simulink model "reglersystem"  (R2017a)
settings: Solver=FixedStepAuto  StartTime=0.0  StopTime=inf  RelTol=1e-3
libraries: robotlib x9, simulink x2
settings Model: Creator=simonpersson  LastModifiedBy=simonpersson
settings OptimizationCC: PassReuseOutputArgsAs=Individual arguments  MaxStackSize=64
settings DebuggingCC: ParameterTunabilityLossMsg=error
settings HardwareCC: ProdBitPerPointer=32  ProdBitPerSizeT=32  ProdBitPerPtrDiffT=32  ProdLargestAtomicFloat=None  ProdIntDivRoundTo=Undefined  ProdEndianess=Unspecified  ProdWordSize=32  ProdHWDeviceType=Generic->Unspecified (assume 32-bit Generic)
settings SFSimCC: MATLABDynamicMemAlloc=off
settings RTWCC: SystemTargetFile=ert.tlc  HardwareBoard=Robot Operating System (ROS)  TLCOptions="-aInlineSetEventsForThisBaseRateFcn=TLC_FALSE -aSuppressMultiTaskScheduler=TLC_FALSE  -aRateBasedStepFcn=0"  TemplateMakefile=ert_default_tmf  Description=Embedded Coder  GenerateReport=on  Toolchain=Catkin  IncludeHyperlinkInReport=on  LaunchReport=on  TargetLang=C++  GenerateTraceInfo=on  GenerateTraceReport=on  GenerateTraceReportSl=on  GenerateTraceReportSf=on  GenerateTraceReportEml=on
settings CodeAppCC: ForceParamTrailComments=on  IgnoreCustomStorageClasses=off  OperatorAnnotations=on  SimulinkDataObjDesc=on  SFDataObjDesc=on  MATLABFcnDesc=on  InsertBlockDesc=on  MATLABSourceComments=on
settings ERTTargetCC: SupportContinuousTime=on

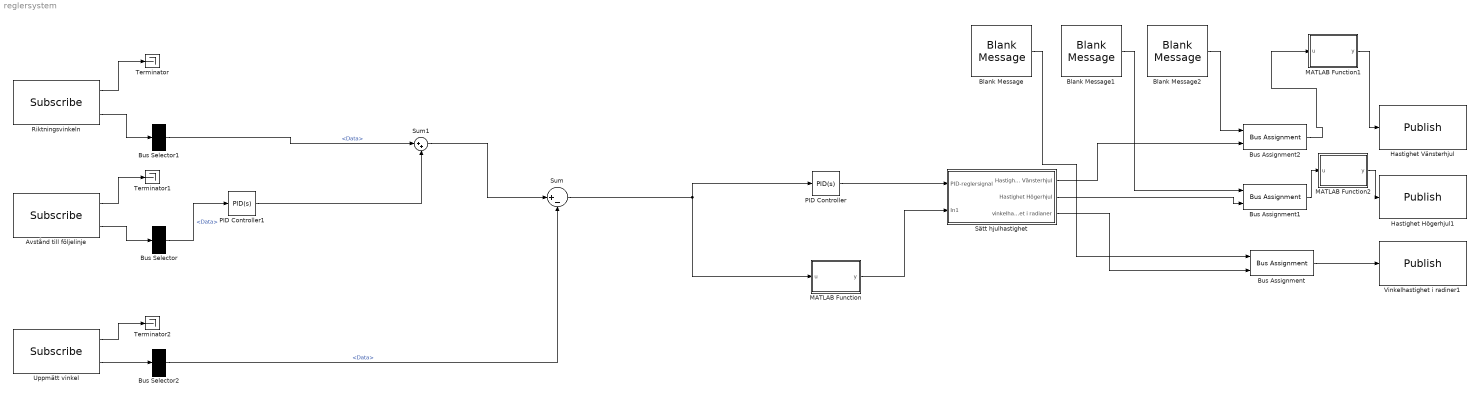
== system reglersystem ==
  Avstånd till följelinje : robotlib/Subscribe  SourceLibraryInfo=This block requires Robotics System Toolbox  topicSource=Specify your own  topic=/distSide_camshifttrack  messageType=std_msgs/Float64  sampleTime=inf  messageQueueLength=1
      settings: SourceProductBaseCode=RO
  Blank Message : robotlib/Blank Message  SourceLibraryInfo=This block requires Robotics System Toolbox  messageType=std_msgs/Float64  SampleTime=inf
      settings: SourceProductBaseCode=RO
  Blank Message1 : robotlib/Blank Message  SourceLibraryInfo=This block requires Robotics System Toolbox  messageType=std_msgs/Float64  SampleTime=inf
      settings: SourceProductBaseCode=RO
  Blank Message2 : robotlib/Blank Message  SourceLibraryInfo=This block requires Robotics System Toolbox  messageType=std_msgs/Float64  SampleTime=inf
      settings: SourceProductBaseCode=RO
  Bus Assignment : BusAssignment  AssignedSignals=Data
  Bus Assignment1 : BusAssignment  AssignedSignals=Data
  Bus Assignment2 : BusAssignment  AssignedSignals=Data
  Bus Selector : BusSelector  OutputSignals=Data
  Bus Selector1 : BusSelector  OutputSignals=Data
  Bus Selector2 : BusSelector  OutputSignals=Data
  Hastighet Högerhjul1 : robotlib/Publish  SourceLibraryInfo=This block requires Robotics System Toolbox  topicSource=Specify your own  topic=/motor_H  messageType=std_msgs/Float64  messageQueueLength=1
      settings: SourceProductBaseCode=RO
  Hastighet Vänsterhjul : robotlib/Publish  SourceLibraryInfo=This block requires Robotics System Toolbox  topicSource=Specify your own  topic=/motor_V  messageType=std_msgs/Float64  messageQueueLength=1
      settings: SourceProductBaseCode=RO
  MATLAB Function : MATLAB Function  TreatAsAtomicUnit=on
  MATLAB Function1 : MATLAB Function  TreatAsAtomicUnit=on
  MATLAB Function2 : MATLAB Function  TreatAsAtomicUnit=on
  PID Controller : simulink/Continuous/PID Controller  Controller=PID  TimeDomain=Continuous-time  SampleTime=-1  IntegratorMethod=Forward Euler  FilterMethod=Forward Euler  Form=Parallel  UseFilter=on  ControllerParametersSource=internal  P=0.380496346065877  I=0.0371695412767303  D=0.374516234293047  N=3.18403469424397  InitialConditionSource=internal  InitialConditionForIntegrator=0  InitialConditionForFilter=0  ExternalReset=none  LimitOutput=off  UpperSaturationLimit=inf  LowerSaturationLimit=-inf  LinearizeAsGain=on  AntiWindupMode=none  Kb=1  TrackingMode=off  Kt=1  PParamMin=[]  PParamMax=[]  IParamMin=[]  IParamMax=[]  DParamMin=[]  DParamMax=[]  NParamMin=[]  NParamMax=[]  KbParamMin=[]  KbParamMax=[]  KtParamMin=[]  KtParamMax=[]  POutMin=[]  POutMax=[]  IOutMin=[]  IOutMax=[]  DOutMin=[]  DOutMax=[]  NOutMin=[]  NOutMax=[]  KbOutMin=[]  KbOutMax=[]  KtOutMin=[]  KtOutMax=[]  IntegratorOutMin=[]  IntegratorOutMax=[]  FilterOutMin=[]  FilterOutMax=[]  SumOutMin=[]  SumOutMax=[]  SumI1OutMin=[]  SumI1OutMax=[]  SumI2OutMin=[]  SumI2OutMax=[]  SumI3OutMin=[]  SumI3OutMax=[]  SumDOutMin=[]  SumDOutMax=[]  SaturationOutMin=[]  SaturationOutMax=[]  IntegratorContinuousStateAttributes=''  IntegratorStateMustResolveToSignalObject=off  IntegratorRTWStateStorageClass=Auto  FilterContinuousStateAttributes=''  FilterStateMustResolveToSignalObject=off  FilterRTWStateStorageClass=Auto  DifferentiatorICPrevScaledInput=0  DifferentiatorOutMin=[]  DifferentiatorOutMax=[]  InitialConditionSetting=State (most efficient)
  PID Controller1 : simulink/Continuous/PID Controller  Controller=PID  TimeDomain=Continuous-time  SampleTime=-1  IntegratorMethod=Forward Euler  FilterMethod=Forward Euler  Form=Parallel  UseFilter=on  ControllerParametersSource=internal  P=-1.19625255559911  I=-0.1605986435679  D=-1.60647701550428  N=1.06418389328725  InitialConditionSource=internal  InitialConditionForIntegrator=0  InitialConditionForFilter=0  ExternalReset=none  LimitOutput=off  UpperSaturationLimit=inf  LowerSaturationLimit=-inf  LinearizeAsGain=on  AntiWindupMode=none  Kb=1  TrackingMode=off  Kt=1  PParamMin=[]  PParamMax=[]  IParamMin=[]  IParamMax=[]  DParamMin=[]  DParamMax=[]  NParamMin=[]  NParamMax=[]  KbParamMin=[]  KbParamMax=[]  KtParamMin=[]  KtParamMax=[]  POutMin=[]  POutMax=[]  IOutMin=[]  IOutMax=[]  DOutMin=[]  DOutMax=[]  NOutMin=[]  NOutMax=[]  KbOutMin=[]  KbOutMax=[]  KtOutMin=[]  KtOutMax=[]  IntegratorOutMin=[]  IntegratorOutMax=[]  FilterOutMin=[]  FilterOutMax=[]  SumOutMin=[]  SumOutMax=[]  SumI1OutMin=[]  SumI1OutMax=[]  SumI2OutMin=[]  SumI2OutMax=[]  SumI3OutMin=[]  SumI3OutMax=[]  SumDOutMin=[]  SumDOutMax=[]  SaturationOutMin=[]  SaturationOutMax=[]  IntegratorContinuousStateAttributes=''  IntegratorStateMustResolveToSignalObject=off  IntegratorRTWStateStorageClass=Auto  FilterContinuousStateAttributes=''  FilterStateMustResolveToSignalObject=off  FilterRTWStateStorageClass=Auto  DifferentiatorICPrevScaledInput=0  DifferentiatorOutMin=[]  DifferentiatorOutMax=[]  InitialConditionSetting=State (most efficient)
  Riktningsvinkeln : robotlib/Subscribe  SourceLibraryInfo=This block requires Robotics System Toolbox  topicSource=Specify your own  topic=/ang__camshifttrack  messageType=std_msgs/Float64  sampleTime=inf  messageQueueLength=1
      settings: SourceProductBaseCode=RO
  Sum : Sum  Inputs=|+-
  Sum1 : Sum  Inputs=|++
  Sätt hjulhastighet : Subsystem
  Terminator : Terminator
  Terminator1 : Terminator
  Terminator2 : Terminator
  Uppmätt vinkel : robotlib/Subscribe  SourceLibraryInfo=This block requires Robotics System Toolbox  topicSource=Specify your own  topic=/heading  messageType=std_msgs/Float64  sampleTime=inf  messageQueueLength=1
      settings: SourceProductBaseCode=RO
  Vinkelhastighet i radiner1 : robotlib/Publish  SourceLibraryInfo=This block requires Robotics System Toolbox  topicSource=Specify your own  topic=/vinkelHastighet  messageType=std_msgs/Float64  messageQueueLength=1
      settings: SourceProductBaseCode=RO
  wires:
  Sätt hjulhastighet/3(vinkelhastighet i radianer) -> Bus Assignment/2
  Sum/1 -> PID Controller/1, MATLAB Function/1(u)
  MATLAB Function/1(y) -> Sätt hjulhastighet/2(In1)
  PID Controller/1 -> Sätt hjulhastighet/1("PID-reglersignal ")
  Sätt hjulhastighet/2(Hastighet Högerhjul) -> Bus Assignment1/2
  Bus Selector2/1 -> Sum/2  "<Data>"
  Sätt hjulhastighet/1(Hastighet Vänsterhjul) -> Bus Assignment2/2
  Sum1/1 -> Sum/1
  PID Controller1/1 -> Sum1/2
  Riktningsvinkeln/1 -> Terminator/1
  Avstånd till följelinje/1 -> Terminator1/1
  Avstånd till följelinje/2 -> Bus Selector/1
  Bus Selector/1 -> PID Controller1/1  "<Data>"
  Riktningsvinkeln/2 -> Bus Selector1/1
  Bus Selector1/1 -> Sum1/1  "<Data>"
  Uppmätt vinkel/2 -> Bus Selector2/1
  Uppmätt vinkel/1 -> Terminator2/1
  Blank Message/1 -> Bus Assignment/1
  Bus Assignment/1 -> Vinkelhastighet i radiner1/1
  Blank Message1/1 -> Bus Assignment1/1
  Blank Message2/1 -> Bus Assignment2/1
  Bus Assignment1/1 -> MATLAB Function2/1(u)
  Bus Assignment2/1 -> MATLAB Function1/1(u)
  MATLAB Function1/1(y) -> Hastighet Vänsterhjul/1
  MATLAB Function2/1(y) -> Hastighet Högerhjul1/1

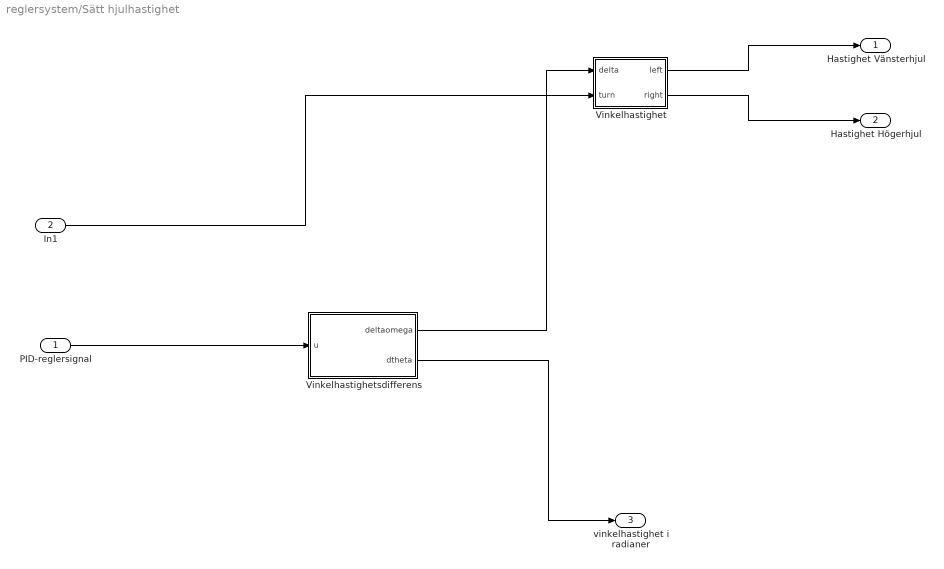
== system reglersystem/Sätt hjulhastighet ==
  "PID-reglersignal " : Inport
  In1 : Inport  Port=2
  Vinkelhastighet : MATLAB Function  TreatAsAtomicUnit=on
  Vinkelhastighetsdifferens : MATLAB Function  TreatAsAtomicUnit=on
  Hastighet Vänsterhjul : Outport  OutDataTypeStr=double
  Hastighet Högerhjul : Outport  Port=2  OutDataTypeStr=double
  vinkelhastighet i radianer : Outport  Port=3  OutDataTypeStr=double
  wires:
  "PID-reglersignal "/1 -> Vinkelhastighetsdifferens/1(u)
  Vinkelhastighetsdifferens/1(deltaomega) -> Vinkelhastighet/1(delta)
  Vinkelhastighetsdifferens/2(dtheta) -> vinkelhastighet i radianer/1
  Vinkelhastighet/1(left) -> Hastighet Vänsterhjul/1
  Vinkelhastighet/2(right) -> Hastighet Högerhjul/1
  In1/1 -> Vinkelhastighet/2(turn)

== matlab function reglersystem/Sätt hjulhastighet/Vinkelhastighet ==
  data: delta input; left output; right output; turn input
function [left,right] = fcn(delta,turn)
r=0.075;
if(turn==0)
if(delta<0)%sväng höger
    left=(1/(2*r*pi))*2*pi;
    right=((1/(2*r*pi))*2*pi)-abs(delta);

else if(delta>0)%sväng vänster
    right=(1/(2*r*pi))*2*pi;
    left=((1/(2*r*pi))*2*pi)-abs(delta); 
    else % kör rakt
    right =(1/(2*r*pi))*2*pi;
    left=(1/(2*r*pi))*2*pi;
    end
end
else if(turn<0)  
    right =(1/(6*r*pi))*2*pi;
    left=-(1/(6*r*pi))*2*pi;
    
    else
        right =-(1/(6*r*pi))*2*pi;
        left=(1/(6*r*pi))*2*pi;
    end
end
end

== matlab function reglersystem/MATLAB Function ==
  data: u input; y output
function y = fcn(u)
%#codegen
if(u>0.7)
    u=1;
else if(u<-0.7)
        u=-1;
else
    u=0;
    end
end

y = u;

== matlab function reglersystem/MATLAB Function1 ==
  data: u input; y output
function y = fcn(u)
y = 11.4474+5.96269 * u;

== matlab function reglersystem/MATLAB Function2 ==
  data: u input; y output
function y = fcn(u)
y = 10.2732+5.41462 * u;

== matlab function reglersystem/Sätt hjulhastighet/Vinkelhastighetsdifferens ==
  data: u input; deltaomega output; dtheta output double
function [deltaomega,dtheta] = fcn(u)
b=0.55; %avstånd mellan hjul
r=0.075; %hjulradie
u=u*360/(2*pi);
z=u;

dtheta=z*2*pi/360;           %robotens vinkelhastighet
deltaomega=((dtheta.*b)./r);         %differensen i vinkelhastighet mellan hjulen
end
